simulink model "TwoLinkPlanarRobotMotionControl"  (Simulink 7.9)
settings: Solver=ode1  StartTime=0.0  StopTime=10.0  FixedStep=0.01  RelTol=1e-3
values from neighbouring files (symbols this model uses):
  m = [1 1]    [FurutaPendulum_Dynamics.m]    (also in Question_2.m = [m_1 m_2]; test_ForwardDynamics.m = [1 1 1]; test_TwoLinkPlanarRobotDynamics.m = [m1 m2]; test_TwoLinkPlanarRobotHybridControl.m = [m1 m2])
  N = 5    [createEllipsoid.m]
  s = tf('s')    [Current_loop_bode.m]    (also in Question_1.m = 15)
undefined symbols (not defined in the file or in its folder): rad
libraries: mblibv1 x14
settings Model: Creator=leavesdown_admin  LastModifiedBy=leavesdown_admin
settings SimMechanicsCC: VisDuringSimulation=on
settings ConfigurationSet: Description=SimMechanics 2G

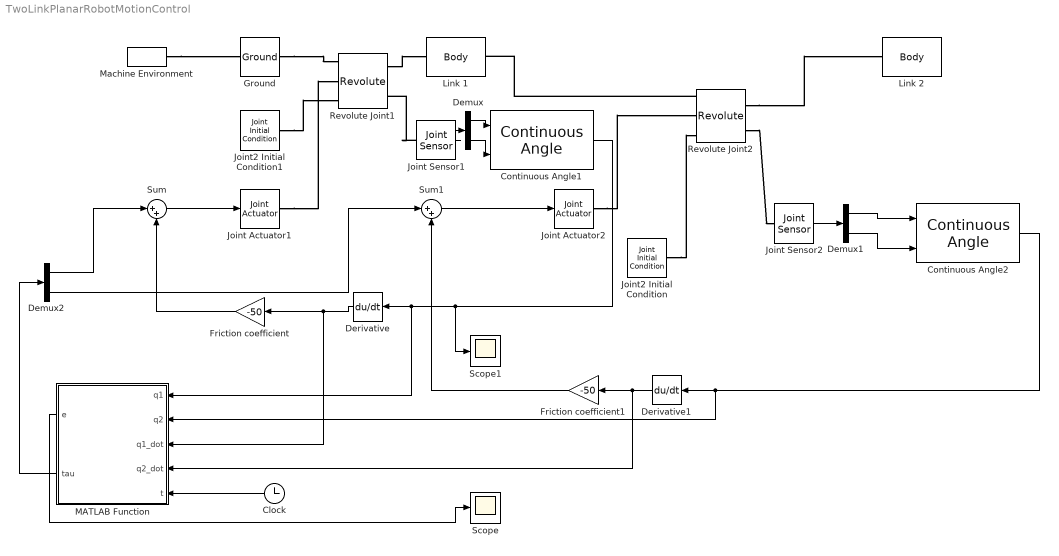
== system TwoLinkPlanarRobotMotionControl ==
  Clock : Clock
  Continuous Angle1 : mblibv1/Utilities/Continuous Angle  rad=rad  rads=rad/s
  Continuous Angle2 : mblibv1/Utilities/Continuous Angle  rad=rad  rads=rad/s
  Demux : Demux  Outputs=2
  Demux1 : Demux  Outputs=2
  Demux2 : Demux  Outputs=2
  Derivative : Derivative
  Derivative1 : Derivative
  Friction coefficient : Gain  Gain=-50
  Friction coefficient1 : Gain  Gain=-50
  Ground : mblibv1/Bodies/Ground  UpdateFromCAD=off  LeftPortType=env  RightPortType=workingframe  PhysicalDomain=Mechanical  DialogClass=GroundBlock  CoordPosition=[0 0 1]  CoordPositionUnits=m  StateVectorMgrId=5  MachineId=[3 0]  ShowEnvPort=on
  Joint Actuator1 : mblibv1/Sensors &  Actuators/Joint Actuator  UpdateFromCAD=off  PhysicalDomain=Mechanical  PortType=blob  ActuationStyle=Force  AngleUnits=deg  ArcVelocityUnits=deg/s  ArcAccelerationUnits=deg/s^2  CoordPositionUnits=m  VelocityUnits=m/s  AccelerationUnits=m/s^2  ForceUnits=N  TorqueUnits=N*m  ActiveIO=on  Width=1  DialogClass=MechanicalActuatorBlock  Primitive=R1  ReferenceFrame=Absolute (World)
  Joint Actuator2 : mblibv1/Sensors &  Actuators/Joint Actuator  UpdateFromCAD=off  PhysicalDomain=Mechanical  PortType=blob  ActuationStyle=Force  AngleUnits=deg  ArcVelocityUnits=deg/s  ArcAccelerationUnits=deg/s^2  CoordPositionUnits=m  VelocityUnits=m/s  AccelerationUnits=m/s^2  ForceUnits=N  TorqueUnits=N*m  ActiveIO=on  Width=1  DialogClass=MechanicalActuatorBlock  Primitive=R1  ReferenceFrame=Absolute (World)
  Joint Sensor1 : mblibv1/Sensors &  Actuators/Joint Sensor  UpdateFromCAD=off  PhysicalDomain=Mechanical  PortType=blob  Muxed=on  Pose=off  Angle=on  AngleUnits=rad  ArcVelocity=on  ArcVelocityUnits=rad/s  ArcAcceleration=off  ArcAccelerationUnits=deg/s^2  CoordPosition=on  CoordPositionUnits=m  Velocity=off  VelocityUnits=m/s  Acceleration=off  AccelerationUnits=m/s^2  Quaternion=on  QuaternionDT=off  QuaternionDDT=off  QuaternionUnits=off  OutputVector=[1]  ActiveIO=on  Width=2  DialogClass=MechanicalSensorBlock  Primitive=R1  Force=off  ForceUnits=N  Torque=off  TorqueUnits=N*m  ReferenceFrame=Absolute (World)  ReactionSensedSide=Base  ReactionReferenceFrame=Absolute (World)  ReactionForce=off  ReactionForceUnits=N  ReactionMoment=off  ReactionMomentUnits=N*m
  Joint Sensor2 : mblibv1/Sensors &  Actuators/Joint Sensor  UpdateFromCAD=off  PhysicalDomain=Mechanical  PortType=blob  Muxed=on  Pose=off  Angle=on  AngleUnits=rad  ArcVelocity=on  ArcVelocityUnits=rad/s  ArcAcceleration=off  ArcAccelerationUnits=deg/s^2  CoordPosition=on  CoordPositionUnits=m  Velocity=off  VelocityUnits=m/s  Acceleration=off  AccelerationUnits=m/s^2  Quaternion=on  QuaternionDT=off  QuaternionDDT=off  QuaternionUnits=off  OutputVector=[1]  ActiveIO=on  Width=2  DialogClass=MechanicalSensorBlock  Primitive=R1  Force=off  ForceUnits=N  Torque=off  TorqueUnits=N*m  ReferenceFrame=Absolute (World)  ReactionSensedSide=Base  ReactionReferenceFrame=Absolute (World)  ReactionForce=off  ReactionForceUnits=N  ReactionMoment=off  ReactionMomentUnits=N*m
  Joint2 Initial Condition : mblibv1/Sensors &  Actuators/Joint Initial Condition  UpdateFromCAD=off  LeftPortType=blob  RightPortType=blob  PhysicalDomain=mechanical  DialogClass=InitialConditionBlock  InitialConditions=P1$false$0$m$deg$0$m/s$deg/s#P2$false$0$m$deg$0$m/s$deg/s#P3$false$0$m$deg$0$m/s$deg/s#R1$true$0$m$rad$0$m/s$rad/s#R2$false$0$m$deg$0$m/s$deg/s#R3$false$0$m$deg$0$m/s$deg/s#S$false$0$m$deg$0$m/s$deg/s  P1PIC=0  P1VIC=0  P2PIC=0  P2VIC=0  P3PIC=0  P3VIC=0  R1PIC=0  R1VIC=0  R2PIC=0  R2VIC=0  R3PIC=0  R3VIC=0  SPIC=0  SVIC=0
  Joint2 Initial Condition1 : mblibv1/Sensors &  Actuators/Joint Initial Condition  UpdateFromCAD=off  LeftPortType=blob  RightPortType=blob  PhysicalDomain=mechanical  DialogClass=InitialConditionBlock  InitialConditions=P1$false$0$m$deg$0$m/s$deg/s#P2$false$0$m$deg$0$m/s$deg/s#P3$false$0$m$deg$0$m/s$deg/s#R1$true$pi/4$m$rad$0$m/s$rad/s#R2$false$0$m$deg$0$m/s$deg/s#R3$false$0$m$deg$0$m/s$deg/s#S$false$0$m$deg$0$m/s$deg/s  P1PIC=0  P1VIC=0  P2PIC=0  P2VIC=0  P3PIC=0  P3VIC=0  R1PIC=pi/4  R1VIC=0  R2PIC=0  R2VIC=0  R3PIC=0  R3VIC=0  SPIC=0  SVIC=0
  Link 1 : mblibv1/Bodies/Body  LConnTagsString=CS1  RConnTagsString=CS2  UpdateFromCAD=off  DialogClass=MechanicalBodyBlock  Mass=50  MassUnits=kg  InertiaUnits=kg*m^2  Inertia=[0 0 0;0 10 0;0 0 10];  Shape=Cylinder  ShapeDims=[1 1]  ShapeUnits=m  ShapeUse=false  Density=1  DensityUnits=kg/m^3  DensityUse=false  GraphicsMode=MACHINE_DEFAULT  BodyColorSelMode=MACHINE_DEFAULT  BodyColor=[1 0 0]  AttachedToCS=CG  CG=Left$CG$[-0.5 0 0]$CS2$CS2$m$eye(3)$3x3 Transform$rad$CS2$false$none  WorkingFrames=Left$CS1$[0 0 0]$Adjoining$Adjoining$m$eye(3)$3x3 Transform$rad$Adjoining$true$none#Right$CS2$[1 0 0]$CS1$CS1$m$eye(3)$3x3 Transform$rad$CS1$true$none  CGPos=[-0.5 0 0]  CGRot=eye(3)  CS0Pos=[]  CS0Rot=[]  CS1Pos=[0 0 0]  CS1Rot=eye(3)  CS2Pos=[1 0 0]  CS2Rot=eye(3)  CS3Pos=[]  CS3Rot=[]  CS4Pos=[]  CS4Rot=[]  CS5Pos=[]  CS5Rot=[]  CS6Pos=[]  CS6Rot=[]  CS7Pos=[]  CS7Rot=[]  CS8Pos=[]  CS8Rot=[]  CS9Pos=[]  CS9Rot=[]  CS10Pos=[]  CS10Rot=[]  CS11Pos=[]  CS11Rot=[]  CS12Pos=[]  CS12Rot=[]  CS13Pos=[]  CS13Rot=[]  CS14Pos=[]  CS14Rot=[]  CS15Pos=[]  CS15Rot=[]  CS16Pos=[]  CS16Rot=[]  CS17Pos=[]  CS17Rot=[]  CS18Pos=[]  CS18Rot=[]  CS19Pos=[]  CS19Rot=[]  CS20Pos=[]  CS20Rot=[]
  Link 2 : mblibv1/Bodies/Body  LConnTagsString=CS1  RConnTagsString=CS2  UpdateFromCAD=off  DialogClass=MechanicalBodyBlock  Mass=50  MassUnits=kg  InertiaUnits=kg*m^2  Inertia=[0 0 0;0 10 0;0 0 10];  Shape=Cylinder  ShapeDims=[1 1]  ShapeUnits=m  ShapeUse=false  Density=1  DensityUnits=kg/m^3  DensityUse=false  GraphicsMode=MACHINE_DEFAULT  BodyColorSelMode=MACHINE_DEFAULT  BodyColor=[1 0 0]  AttachedToCS=CG  CG=Left$CG$[-0.5 0 0]$CS2$CS2$m$eye(3)$3x3 Transform$rad$CS2$false$none  WorkingFrames=Left$CS1$[0 0 0]$Adjoining$Adjoining$m$eye(3)$3x3 Transform$rad$Adjoining$true$none#Right$CS2$[1 0 0]$CS1$CS1$m$eye(3)$3x3 Transform$rad$CS1$true$none  CGPos=[-0.5 0 0]  CGRot=eye(3)  CS0Pos=[]  CS0Rot=[]  CS1Pos=[0 0 0]  CS1Rot=eye(3)  CS2Pos=[1 0 0]  CS2Rot=eye(3)  CS3Pos=[]  CS3Rot=[]  CS4Pos=[]  CS4Rot=[]  CS5Pos=[]  CS5Rot=[]  CS6Pos=[]  CS6Rot=[]  CS7Pos=[]  CS7Rot=[]  CS8Pos=[]  CS8Rot=[]  CS9Pos=[]  CS9Rot=[]  CS10Pos=[]  CS10Rot=[]  CS11Pos=[]  CS11Rot=[]  CS12Pos=[]  CS12Rot=[]  CS13Pos=[]  CS13Rot=[]  CS14Pos=[]  CS14Rot=[]  CS15Pos=[]  CS15Rot=[]  CS16Pos=[]  CS16Rot=[]  CS17Pos=[]  CS17Rot=[]  CS18Pos=[]  CS18Rot=[]  CS19Pos=[]  CS19Rot=[]  CS20Pos=[]  CS20Rot=[]
  MATLAB Function : MATLAB Function  TreatAsAtomicUnit=on
  Machine Environment : mblibv1/Bodies/Machine Environment  PortType=env  PhysicalDomain=Mechanical  DialogTemplateClass=MECH.MachineEnvironment  SyncWhenCopied=off  Gravity=[0 -9.81 0]  GravityUnits=m/s^2  GravityAsSignal=off  Dimensionality=Auto-detect  AnalysisType=Forward dynamics  LinearAssemblyTolerance=1e-3  LinearAssemblyToleranceUnits=m  AngularAssemblyTolerance=1e-3  AngularAssemblyToleranceUnits=rad  ConstraintSolverType=Stabilizing  ConstraintRelTolerance=1e-4  ConstraintAbsTolerance=1e-4  UseRobustSingularityHandling=off  RedundancyAnalysisToleranceType=Automatically select tolerance  RedundancyAnalysisTolerance=1e-14  StatePerturbationType=Fixed  PerturbationSize=1e-5  VisualizeMachine=on  BodyVisualizationType=Use model default body geometries  BodyColorSelMode=Use model default  DefaultBodyColor=[1 0 0]
  Revolute Joint1 : mblibv1/Joints/Revolute  LConnTagsString=__newl0|SA1|SA2  RConnTagsString=__newr0|SA1  UpdateFromCAD=off  NumSAPorts=3  CutJoint=off  MarkAsCut=off  Primitives=prismatic  PrimitiveProps=R1$Base$[0 0 1]$revolute  DialogClass=JointBlock  R1Axis=[0 0 1]
  Revolute Joint2 : mblibv1/Joints/Revolute  LConnTagsString=__newl0|SA1|SA2  RConnTagsString=__newr0|SA1  UpdateFromCAD=off  NumSAPorts=3  CutJoint=off  MarkAsCut=off  Primitives=prismatic  PrimitiveProps=R1$Base$[0 0 1]$revolute  DialogClass=JointBlock  R1Axis=[0 0 1]
  Scope : Scope
  Scope1 : Scope
      settings: YMin=0.7  YMax=2.4
  Sum : Sum  Inputs=|++
  Sum1 : Sum  Inputs=|++
  wires:
  Sum/1 -> Joint Actuator1/1
  Friction coefficient/1 -> Sum/2
  Sum1/1 -> Joint Actuator2/1
  Friction coefficient1/1 -> Sum1/2
  Derivative1/1 -> Friction coefficient1/1, MATLAB Function/4(q2_dot)
  Derivative/1 -> Friction coefficient/1, MATLAB Function/3(q1_dot)
  Joint Sensor1/1 -> Demux/1
  Demux/1 -> Continuous Angle1/1
  Demux/2 -> Continuous Angle1/2
  Continuous Angle1/1 -> Derivative/1, MATLAB Function/1(q1), Scope1/1
  Joint Sensor2/1 -> Demux1/1
  Demux1/1 -> Continuous Angle2/1
  Demux1/2 -> Continuous Angle2/2
  Continuous Angle2/1 -> Derivative1/1, MATLAB Function/2(q2)
  Clock/1 -> MATLAB Function/5(t)
  MATLAB Function/2(tau) -> Demux2/1
  Demux2/1 -> Sum/1
  Demux2/2 -> Sum1/1
  MATLAB Function/1(e) -> Scope/1
  connections:
  Ground/RConn1 -- Revolute Joint1/LConn1
  Revolute Joint1/RConn1 -- Link 1/LConn1
  Machine Environment/RConn1 -- Ground/LConn1
  Revolute Joint2/LConn1 -- Link 1/RConn1
  Revolute Joint2/RConn1 -- Link 2/LConn1
  Joint Sensor1/LConn1 -- Revolute Joint1/RConn2
  Revolute Joint2/RConn2 -- Joint Sensor2/LConn1
  Joint Actuator1/RConn1 -- Revolute Joint1/LConn2
  Joint Actuator2/RConn1 -- Revolute Joint2/LConn2
  Joint2 Initial Condition/RConn1 -- Revolute Joint2/LConn3
  Joint2 Initial Condition1/RConn1 -- Revolute Joint1/LConn3

== matlab function MATLAB Function ==
  data: e output double; q1 input double; tau output double; q2 input double; q1_dot input double; q2_dot input double; t input double
function [e,tau] = fcn(q1,q2,q1_dot,q2_dot,t)
coder.extrinsic('Newton_Euler_Iteration');

q=[q1;q2];
q_dot=[q1_dot;q2_dot];
Jtype=[0;0];
    a1=1;a2=1;
    n=2;%number of joints
    m1=50;m2=50;
    m=[m1 m2]; %define mass constants
    Il1=10;Il2=10;
    I=zeros(3,3,2);
    I(:,:,1)=[0 0 0;0 Il1 0;0 0 Il1];I(:,:,2)=[0 0 0;0 Il2 0;0 0 Il2];%define inertia tensor
    l1=0.5;l2=0.5;
    r_C=[[l1-a1;0;0] [l2-a2;0;0]];%define com coordinates of each link
    kv=[50;50];%define viscous friction constants
    g=9.8;
    g0=[0;-g;0];%define gravity vector
    DH=[[0;q1;a1;0] [0;q2;a2;0]];
    B=zeros(2,2);
    for i=1:n
        q_ddot_temp=[0;0];
        q_ddot_temp(i)=1;
        B(:,i) = Newton_Euler_Iteration(DH, m, I, r_C, Jtype, [0;0], q_ddot_temp, [0;0;0]);
    end
    Coriolis_Gravity=zeros(2,1);
    Coriolis_Gravity=Newton_Euler_Iteration(DH, m, I, r_C, Jtype, q_dot, [0;0], g0);%compute C(q,\dot{q})\dot{q}+G(q)
    qd=[pi/2-pi/4*cos(2*pi/2*t);pi/4*sin(2*pi/2*t)];
    qd_dot=[pi/4*2*pi/2*sin(2*pi/2*t);pi/4*2*pi/2*cos(2*pi/2*t)];
    qd_ddot=[pi/4*((2*pi/2)^2)*cos(2*pi/2*t);-pi/4*((2*pi/2)^2)*sin(2*pi/2*t)];
    e=q-qd;
    e_dot=q_dot-qd_dot;
    Kp=25.*eye(2);Kd=5.*eye(2);
    tau=-B*Kp*e-B*Kd*e_dot+Coriolis_Gravity+kv.*q_dot+B*qd_ddot;
